simulink model "Simulacion_Resonante"  (R2023a)
settings: Solver=VariableStepAuto  StartTime=0.0  StopTime=4/Frequency  RelTol=1e-3
undefined symbols (not defined in the file): C, Frequency, L, R, Vs
libraries: spsFourierLib x8, spsSeriesRLCBranchLib x7, spsMultimeterLib x2, spsACVoltageSourceLib x2, spsCurrentMeasurementLib x1, sps_lib x1
settings Model: Creator=XIOMARA  LastModifiedBy=Juan Esteban

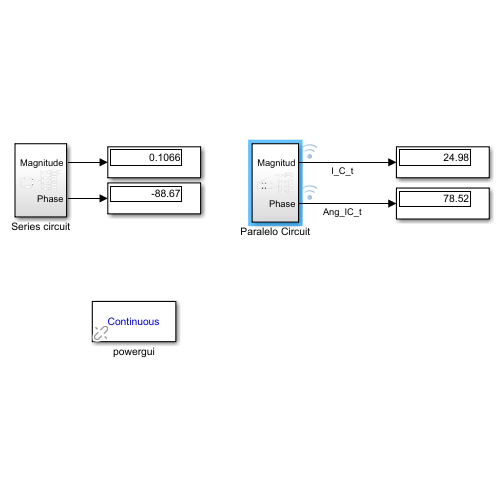
[thumbnail: Simulink's stored preview of the top-level diagram]
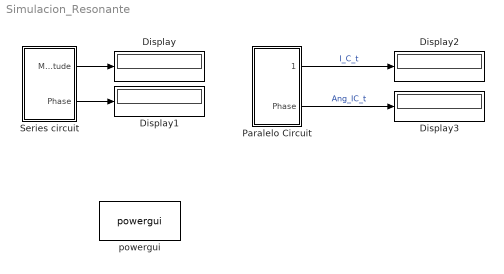
== system Simulacion_Resonante ==
  Display{,1..3} (4 alike) : Display
  Paralelo Circuit : Subsystem
  Series circuit : Subsystem
  powergui : sps_lib/powergui  Priority=1  SimulationMode=Continuous  SampleTime=50e-6  frequency=60  Iterations=50  frequencyindice=1000000  Pbase=100e6  ErrMax=1e-4  UnitsV=kV  UnitsW=MW  buscounter=0  FunctionMessages=off  echomessages=off  EnableUseOfTLC=off  CurrentSourceSwitches=off  DisableSnubberDevices=off  DisableRonSwitches=off  DisableVfSwitches=off  DisplayEquations=off  AutomaticDiscreteSolvers=off  SolverType=Tustin/Backward Euler (TBE)  Interpol=off  ExternalGateDelay=off  methode=off  Ts=100  x0status=blocks  SPID=on  SwTol=0  HookPort=off  NonlinearTolerance=1e-4  nMaxIteration=100  ContinueOnMaxIteration=off  RestoreLinks=warning  ResistiveCurrentMeasurement=off  Frange=[0:2:500]  Ylog=off  Xlog=on  ShowGrid=off  save=off  variable=ZData  structure=0  ZoomFFT=off  StartTime=0.0  cycles=1  DisplayStyle=1  fundamental=60  FreqAxis=off  MaxFrequency=1000  frequencyindicesteady=1  RmsSteady=1  display=off
  wires:
  Series circuit/1(Magnitude) -> Display/1
  Series circuit/2(Phase) -> Display1/1
  Paralelo Circuit/2(Phase) -> Display3/1  "Ang_IC_t"
  Paralelo Circuit/1(Magnitud) -> Display2/1  "I_C_t"

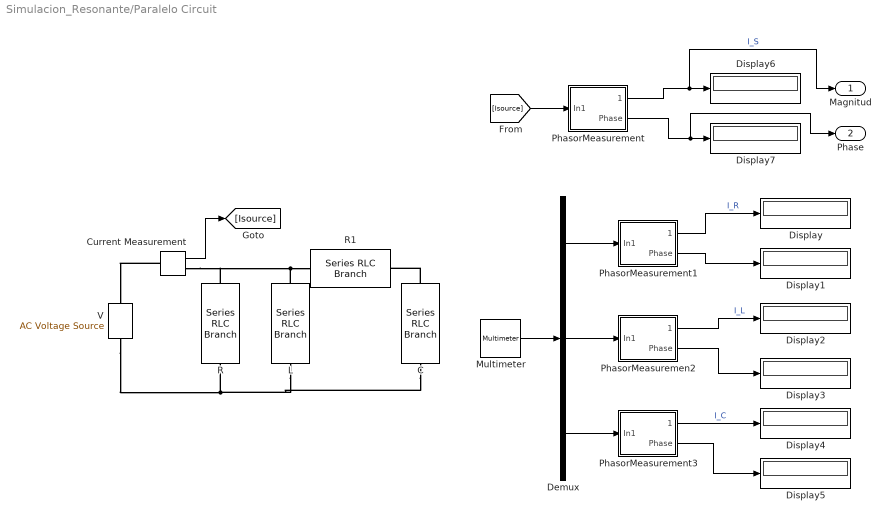
== system Simulacion_Resonante/Paralelo Circuit ==
  " L" : spsSeriesRLCBranchLib/Series RLC Branch  LConnTagsString=__new0  RConnTagsString=__new0  BranchType=L  Resistance=1  Inductance=L  SetiL0=off  InitialCurrent=0  Capacitance=1e-6  Setx0=off  InitialVoltage=0  Measurements=Branch current
  " R1" : spsSeriesRLCBranchLib/Series RLC Branch  LConnTagsString=__new0  RConnTagsString=__new0  BranchType=R  Resistance=1e-4  Inductance=1e-3  SetiL0=off  InitialCurrent=0  Capacitance=1e-6  Setx0=off  InitialVoltage=0  Measurements=None
  "C " : spsSeriesRLCBranchLib/Series RLC Branch  LConnTagsString=__new0  RConnTagsString=__new0  BranchType=C  Resistance=1  Inductance=1e-3  SetiL0=off  InitialCurrent=0  Capacitance=C  Setx0=off  InitialVoltage=0  Measurements=Branch current
  Current Measurement : spsCurrentMeasurementLib/Current Measurement  PhasorSimulation=off  OutputType=Complex  PSBequivalent=0
  Demux : Demux  Outputs=3
  Display{,1..7} (8 alike) : Display
  Multimeter : spsMultimeterLib/Multimeter  L=7  sel=[6 4 5]  yselected={}  Gain=[1 1 1]  OutputType=Complex  PlotAtSimulationStop=off  PhasorSimulation=off
  PhasorMeasuremen2 : Subsystem
  PhasorMeasurement : Subsystem
  PhasorMeasurement1 : Subsystem
  PhasorMeasurement3 : Subsystem
  R : spsSeriesRLCBranchLib/Series RLC Branch  LConnTagsString=__new0  RConnTagsString=__new0  BranchType=R  Resistance=R  Inductance=1e-3  SetiL0=off  InitialCurrent=0  Capacitance=1e-6  Setx0=off  InitialVoltage=0  Measurements=Branch current
  V : spsACVoltageSourceLib/AC Voltage Source  Amplitude=Vs*sqrt(2)  Phase=0  Frequency=Frequency  SampleTime=0  Measurements=None  BusType=swing  Pref=10e3  Qref=0  Qmin=-inf  Qmax=+inf
  Magnitud : Outport
  Phase : Outport  Port=2
  wires:
  Current Measurement/1 -> [Isource]
  PhasorMeasurement1/1(Magnitud) -> Display/1  "I_R"
  PhasorMeasurement1/2(Phase) -> Display1/1
  PhasorMeasuremen2/1(Magnitud) -> Display2/1  "I_L"
  PhasorMeasuremen2/2(Phase) -> Display3/1
  Demux/2 -> PhasorMeasuremen2/1(In1)
  PhasorMeasurement3/1(Magnitud) -> Display4/1  "I_C"
  PhasorMeasurement3/2(Phase) -> Display5/1
  Demux/3 -> PhasorMeasurement3/1(In1)
  Demux/1 -> PhasorMeasurement1/1(In1)
  Multimeter/1 -> Demux/1
  PhasorMeasurement/1(Magnitud) -> Magnitud/1, Display6/1  "I_S"
  [Isource] -> PhasorMeasurement/1(In1)
  PhasorMeasurement/2(Phase) -> Phase/1, Display7/1
  connections:
  " L"/LConn1 -- Current Measurement/RConn1 -- R/LConn1 -- " R1"/RConn1
  Current Measurement/LConn1 -- V/RConn1
  V/LConn1 -- "C "/RConn1 -- " L"/RConn1 -- R/RConn1
  "C "/LConn1 -- " R1"/LConn1

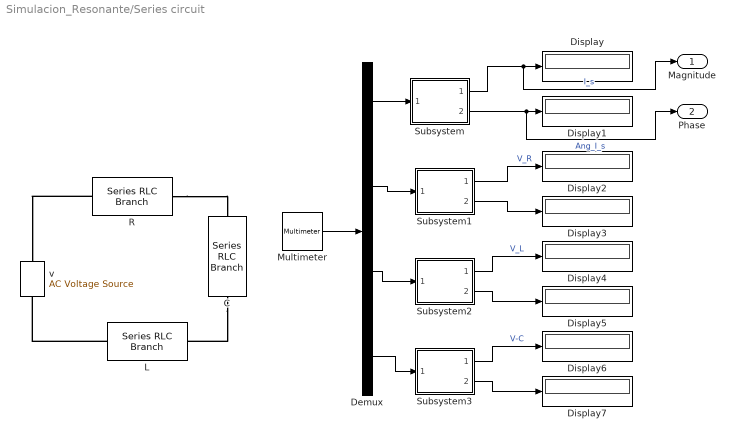
== system Simulacion_Resonante/Series circuit ==
  "C " : spsSeriesRLCBranchLib/Series RLC Branch  LConnTagsString=__new0  RConnTagsString=__new0  BranchType=C  Resistance=1  Inductance=1e-3  SetiL0=off  InitialCurrent=0  Capacitance=C  Setx0=off  InitialVoltage=0  Measurements=Branch voltage
  Demux : Demux
  Display{,1..7} (8 alike) : Display
  L : spsSeriesRLCBranchLib/Series RLC Branch  LConnTagsString=__new0  RConnTagsString=__new0  BranchType=L  Resistance=1  Inductance=L  SetiL0=off  InitialCurrent=0  Capacitance=1e-6  Setx0=off  InitialVoltage=0  Measurements=Branch voltage
  Multimeter : spsMultimeterLib/Multimeter  L=7  sel=[7 3 2 1]  yselected={}  Gain=[1 1 1 1]  OutputType=Complex  PlotAtSimulationStop=off  PhasorSimulation=off
  R : spsSeriesRLCBranchLib/Series RLC Branch  LConnTagsString=__new0  RConnTagsString=__new0  BranchType=R  Resistance=R  Inductance=1e-3  SetiL0=off  InitialCurrent=0  Capacitance=1e-6  Setx0=off  InitialVoltage=0  Measurements=Branch voltage and current
  Subsystem : Subsystem
  Subsystem1 : Subsystem
  Subsystem2 : Subsystem
  Subsystem3 : Subsystem
  v : spsACVoltageSourceLib/AC Voltage Source  Amplitude=Vs*sqrt(2)  Phase=0  Frequency=Frequency  SampleTime=0  Measurements=None  BusType=swing  Pref=10e3  Qref=0  Qmin=-inf  Qmax=+inf
  Magnitude : Outport
  Phase : Outport  Port=2
  wires:
  Subsystem2/1(Magnitude) -> Display4/1  "V_L"
  Subsystem/2(Phase) -> Phase/1, Display1/1  "Ang_I_s"
  Subsystem1/1(Magnitude) -> Display2/1  "V_R"
  Demux/2 -> Subsystem1/1(Signal)
  Subsystem2/2(Phase) -> Display5/1
  Subsystem3/1(Magnitude) -> Display6/1  "V-C"
  Subsystem/1(Magnitude) -> Magnitude/1, Display/1  "I_s"
  Demux/1 -> Subsystem/1(Signal)
  Subsystem1/2(Phase) -> Display3/1
  Demux/4 -> Subsystem3/1(Signal)
  Demux/3 -> Subsystem2/1(Signal)
  Subsystem3/2(Phase) -> Display7/1
  Multimeter/1 -> Demux/1
  connections:
  R/LConn1 -- v/RConn1
  R/RConn1 -- "C "/LConn1
  "C "/RConn1 -- L/RConn1
  L/LConn1 -- v/LConn1

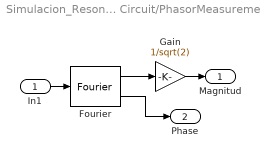
== system Simulacion_Resonante/Paralelo Circuit/PhasorMeasuremen2 ==
  In1 : Inport
  Fourier : spsFourierLib/Fourier  Freq=Frequency  n=1  InInit=[0, 0]  Ts=0
  Gain : Gain  Gain=1/sqrt(2)
  Magnitud : Outport
  Phase : Outport  Port=2
  wires:
  In1/1 -> Fourier/1
  Fourier/1 -> Gain/1
  Gain/1 -> Magnitud/1
  Fourier/2 -> Phase/1

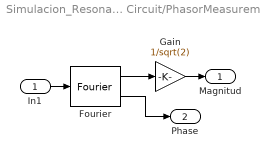
== system Simulacion_Resonante/Paralelo Circuit/PhasorMeasurement ==
  In1 : Inport
  Fourier : spsFourierLib/Fourier  Freq=Frequency  n=1  InInit=[0, 0]  Ts=0
  Gain : Gain  Gain=1/sqrt(2)
  Magnitud : Outport
  Phase : Outport  Port=2
  wires:
  In1/1 -> Fourier/1
  Fourier/1 -> Gain/1
  Gain/1 -> Magnitud/1
  Fourier/2 -> Phase/1

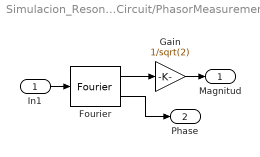
== system Simulacion_Resonante/Paralelo Circuit/PhasorMeasurement1 ==
  In1 : Inport
  Fourier : spsFourierLib/Fourier  Freq=Frequency  n=1  InInit=[0, 0]  Ts=0
  Gain : Gain  Gain=1/sqrt(2)
  Magnitud : Outport
  Phase : Outport  Port=2
  wires:
  In1/1 -> Fourier/1
  Fourier/1 -> Gain/1
  Gain/1 -> Magnitud/1
  Fourier/2 -> Phase/1

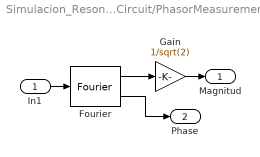
== system Simulacion_Resonante/Paralelo Circuit/PhasorMeasurement3 ==
  In1 : Inport
  Fourier : spsFourierLib/Fourier  Freq=Frequency  n=1  InInit=[0, 0]  Ts=0
  Gain : Gain  Gain=1/sqrt(2)
  Magnitud : Outport
  Phase : Outport  Port=2
  wires:
  In1/1 -> Fourier/1
  Fourier/1 -> Gain/1
  Gain/1 -> Magnitud/1
  Fourier/2 -> Phase/1

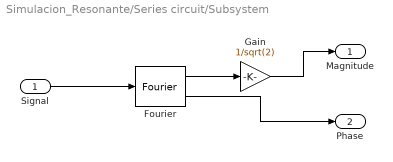
== system Simulacion_Resonante/Series circuit/Subsystem ==
  Signal : Inport
  Fourier : spsFourierLib/Fourier  Freq=Frequency  n=1  InInit=[0, 0]  Ts=0
  Gain : Gain  Gain=1/sqrt(2)
  Magnitude : Outport
  Phase : Outport  Port=2
  wires:
  Fourier/1 -> Gain/1
  Gain/1 -> Magnitude/1
  Signal/1 -> Fourier/1
  Fourier/2 -> Phase/1

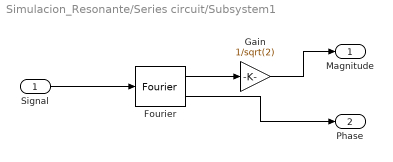
== system Simulacion_Resonante/Series circuit/Subsystem1 ==
  Signal : Inport
  Fourier : spsFourierLib/Fourier  Freq=Frequency  n=1  InInit=[0, 0]  Ts=0
  Gain : Gain  Gain=1/sqrt(2)
  Magnitude : Outport
  Phase : Outport  Port=2
  wires:
  Fourier/1 -> Gain/1
  Gain/1 -> Magnitude/1
  Signal/1 -> Fourier/1
  Fourier/2 -> Phase/1

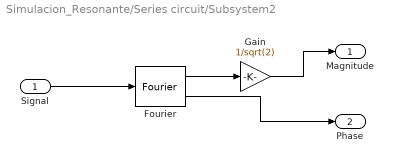
== system Simulacion_Resonante/Series circuit/Subsystem2 ==
  Signal : Inport
  Fourier : spsFourierLib/Fourier  Freq=Frequency  n=1  InInit=[0, 0]  Ts=0
  Gain : Gain  Gain=1/sqrt(2)
  Magnitude : Outport
  Phase : Outport  Port=2
  wires:
  Fourier/1 -> Gain/1
  Gain/1 -> Magnitude/1
  Signal/1 -> Fourier/1
  Fourier/2 -> Phase/1

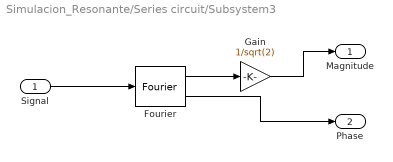
== system Simulacion_Resonante/Series circuit/Subsystem3 ==
  Signal : Inport
  Fourier : spsFourierLib/Fourier  Freq=Frequency  n=1  InInit=[0, 0]  Ts=0
  Gain : Gain  Gain=1/sqrt(2)
  Magnitude : Outport
  Phase : Outport  Port=2
  wires:
  Fourier/1 -> Gain/1
  Gain/1 -> Magnitude/1
  Signal/1 -> Fourier/1
  Fourier/2 -> Phase/1
